simulink subsystem "Engine_Dynamics"  (R2024b)
settings: Solver=VariableStepAuto  StartTime=0.0  StopTime=10.0  RelTol=1e-3
settings Model: Creator=The MathWorks, Inc.  LastModifiedBy=The MathWorks, Inc.

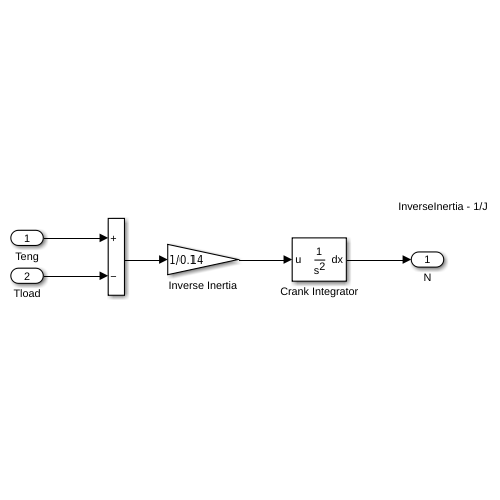
[thumbnail: Simulink's stored preview of the top-level diagram]
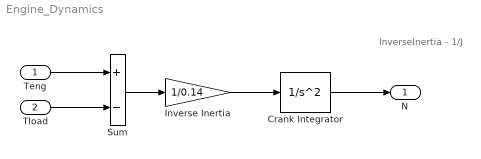
== system Engine_Dynamics ==
  note: InverseInertia - 1/J
  Teng : Inport
  Tload : Inport  Port=2
  Crank Integrator : SecondOrderIntegrator  ICX=0  StateNameX='CrankAngle'  ICDXDT=209.48  StateNameDXDT='CrankAngleVelocity'  ShowOutput=dxdt
  Inverse Inertia : Gain  Gain=1/0.14  SaturateOnIntegerOverflow=on  OutDataTypeStr=Inherit: Same as input  ParamDataTypeStr=Inherit: Same as input
  Sum : Sum  Inputs=+-  InputSameDT=on  SaturateOnIntegerOverflow=on  OutDataTypeStr=Inherit: Same as first input
  N : Outport  Unit=rad/sec  InitialOutput=0  VectorParamsAs1DForOutWhenUnconnected=off
  wires:
  Tload/1 -> Sum/2
  Teng/1 -> Sum/1
  Sum/1 -> Inverse Inertia/1
  Inverse Inertia/1 -> Crank Integrator/1
  Crank Integrator/1 -> N/1
